simulink model "drm_simu"  (Simulink 8.6)
settings: Solver=VariableStepDiscrete  SolverMode=MultiTasking  StartTime=0.0  StopTime=12  RelTol=1e-3
PostLoadFcn:
  | init_drm
values from neighbouring files (symbols this model uses):
  sCRC_poly = struct(     'G16' ,{[1 0 0 0 1 0 0 0 0 0 0 1 0 0 0 0 1] ones(1,16)},     'G8'  ,{[1 0 0 0 1 1 1 0 1] ones(1,8)},     'G6'  ,{[1 1 0 1 1 1 1] ones(1,6)},     'G5'  ,{[1 1 0 1 1 1] ones(1,5)},     'G3'  ,{[1 0 1 0] ones(1,3)},     'G2'  ,{[1 1 1] ones(1,2)},     'G1'  ,{[1 1] 1} )    [crc_poly.m]
undefined symbols (not defined in the file or in its folder): channel, dfilt, fac, get, hot, if_mod, jet, magnitude, msc, ofdm, scrambler, sdc, sFFT, sync
libraries: dspmtrx3 x11, dspstat3 x7, commseqgen2 x6, dspobslib x6, dspsigops x5, commblkintrlv2 x4, dspsrcs4 x4, commsink2 x3, commrandsrc2 x3, commcrc2 x2, commcnvcod2 x2, commsequence2 x2
(part 1 of 2)
settings Model: Creator=Kevin Döring  LastModifiedBy=dtdsv
settings DataIOCC: LimitDataPoints=off  SaveOutput=off  SignalLogging=off  SaveTime=off
settings OptimizationCC: SimCompilerOptimization=on
settings DebuggingCC: InheritedTsInSrcMsg=none  MultiTaskCondExecSysMsg=none  MultiTaskRateTransMsg=warning  FcnCallInpInsideContextMsg=UseLocalSettings  FrameProcessingCompatibilityMsg=none
settings GRTTargetCC: GeneratePreprocessorConditionals=Use local settings

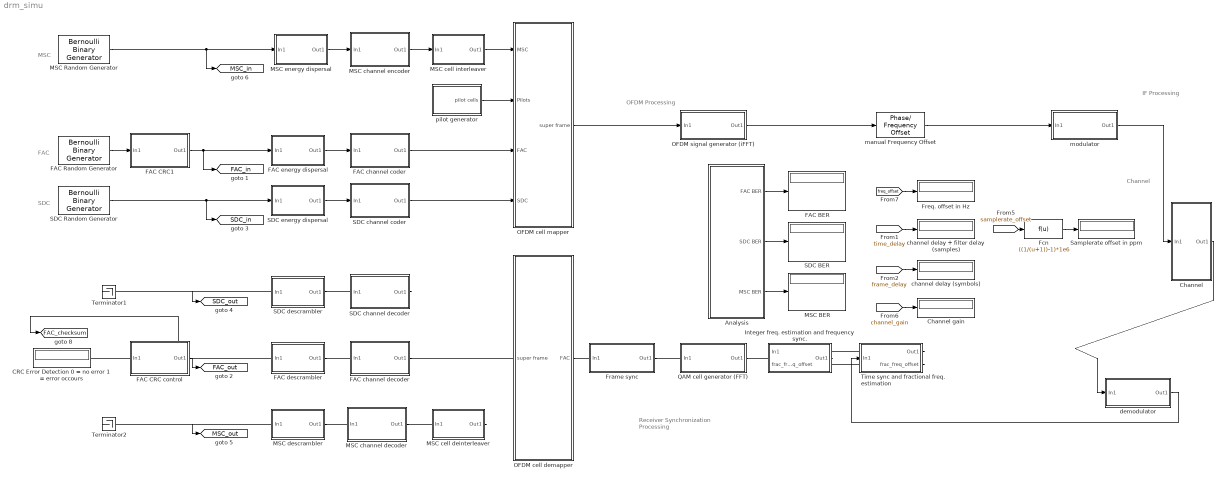
== system drm_simu ==
  note: FAC
  note: SDC
  note: MSC
  note: Receiver
      | Synchronization
      | Processing
  note: IF
      | Processing
  note: OFDM
      | Processing
  note: Channel
  Analysis : Subsystem
  CRC Error Detection 0 = no error 1 = error occours : Display
  Channel : Subsystem
  Channel gain : Display
  FAC BER : Display
  FAC CRC control : Subsystem
  FAC CRC1 : Subsystem
  FAC Random Generator : commrandsrc2/Bernoulli Binary Generator  P=0.5  seed=61  Ts=-1  frameBased=on  sampPerFrame=fac.Nmb_input_bits-8  orient=off  outDataType=double
  FAC channel coder : Subsystem
  FAC channel decoder : Subsystem
  FAC descrambler : Subsystem
  FAC energy dispersal : Subsystem
  Fcn : Fcn  Expr=((1/(u+1))-1)*1e6
  Frame sync : Subsystem
  Freq. offset in Hz : Display
  Integer freq. estimation and frequency sync. : Subsystem
  MSC BER : Display
  MSC Random Generator : commrandsrc2/Bernoulli Binary Generator  P=0.5  seed=61  Ts=sFFT.input_samplerate  frameBased=on  sampPerFrame=msc.Nmb_input_bits  orient=off  outDataType=double
  MSC cell deinterleaver : Subsystem
  MSC cell interleaver : Subsystem
  MSC channel decoder : Subsystem  BlockChoice=4QAM
      settings: AttributesFormatString=%<BlockChoice>  TemplateBlock=MSC_decoder_lib/MSC channel decoder  MemberBlocks=16QAM,4QAM,64QAM
  MSC channel encoder : Subsystem  BlockChoice=4QAM
      settings: AttributesFormatString=%<BlockChoice>  TemplateBlock=MSC_coder_lib/MSC channel encoder  MemberBlocks=16QAM,4QAM,64QAM
  MSC descrambler : Subsystem
  MSC energy dispersal : Subsystem
  OFDM cell demapper : Subsystem
  OFDM cell mapper : Subsystem
  OFDM signal generator (iFFT) : Subsystem
  QAM cell generator (FFT) : Subsystem
  SDC BER : Display
  SDC Random Generator : commrandsrc2/Bernoulli Binary Generator  P=0.5  seed=61  Ts=-1  frameBased=on  sampPerFrame=sdc.Nmb_input_bits  orient=off  outDataType=double
  SDC channel coder : Subsystem  BlockChoice=4QAM
      settings: AttributesFormatString=%<BlockChoice>  TemplateBlock=SDC_coder_lib/SDC channel coder  MemberBlocks=16QAM,4QAM
  SDC channel decoder : Subsystem  BlockChoice=4QAM
      settings: AttributesFormatString=%<BlockChoice>  TemplateBlock=SDC_decoder_lib/SDC channel decoder  MemberBlocks=16QAM,4QAM
  SDC descrambler : Subsystem
  SDC energy dispersal : Subsystem
  Samplerate offset in ppm : Display
  Terminator1 : Terminator
  Terminator2 : Terminator
  Time sync and fractional freq. estimation : Subsystem
  channel delay (symbols) : Display
  channel delay + filter delay (samples) : Display
  demodulator : Subsystem
  manual Frequency Offset : commrflib2/Phase// Frequency Offset  phaseOffset=0  freqPort=off  freqOffset=0
  modulator : Subsystem
  pilot generator : Subsystem
  tag scope: FAC_checksum=global, FAC_in=global, FAC_out=global, MSC_in=global, MSC_out=global, SDC_in=global, SDC_out=global
  wires:
  FAC Random Generator/1 -> FAC CRC1/1(In1)
  FAC energy dispersal/1(Out1) -> FAC channel coder/1(In1)
  FAC descrambler/1(Out1) -> [FAC_out], FAC CRC control/1(In1)
  FAC CRC1/1(Out1) -> FAC energy dispersal/1(In1), [FAC_in]
  FAC channel decoder/1(Out1) -> FAC descrambler/1(In1)
  FAC CRC control/1(Out1) -> CRC Error Detection 0 = no error 1 = error occours/1, [FAC_checksum]
  pilot generator/1(pilot cells) -> OFDM cell mapper/2(Pilots)
  SDC Random Generator/1 -> SDC energy dispersal/1(In1), [SDC_in]
  SDC energy dispersal/1(Out1) -> SDC channel coder/1(In1)
  SDC channel decoder/1(Out1) -> SDC descrambler/1(In1)
  SDC channel coder/1(Out1) -> OFDM cell mapper/4(SDC)
  SDC descrambler/1(Out1) -> [SDC_out], Terminator1/1
  FAC channel coder/1(Out1) -> OFDM cell mapper/3(FAC)
  ? -> SDC channel decoder/1(In1)
  MSC Random Generator/1 -> MSC energy dispersal/1(In1), [MSC_in]
  MSC channel encoder/1(Out1) -> MSC cell interleaver/1(In1)
  MSC energy dispersal/1(Out1) -> MSC channel encoder/1(In1)
  MSC cell interleaver/1(Out1) -> OFDM cell mapper/1(MSC)
  MSC channel decoder/1(Out1) -> MSC descrambler/1(In1)
  MSC cell deinterleaver/1(Out1) -> MSC channel decoder/1(In1)
  MSC descrambler/1(Out1) -> Terminator2/1, [MSC_out]
  ? -> MSC cell deinterleaver/1(In1)
  OFDM cell mapper/1(super frame) -> OFDM signal generator (iFFT)/1(In1)
  Analysis/2(SDC BER) -> SDC BER/1
  Analysis/3(MSC BER) -> MSC BER/1
  Analysis/1(FAC BER) -> FAC BER/1
  Frame sync/1(Out1) -> OFDM cell demapper/1(super frame)
  OFDM signal generator (iFFT)/1(Out1) -> manual Frequency Offset/1
  OFDM cell demapper/1(FAC) -> FAC channel decoder/1(In1)
  [freq_offset] -> Freq. offset in Hz/1
  [channel_gain] -> Channel gain/1
  [time_delay] -> channel delay + filter delay (samples)/1
  [frame_delay] -> channel delay (symbols)/1
  modulator/1(Out1) -> Channel/1(In1)
  [samplerate_offset] -> Fcn/1
  Fcn/1 -> Samplerate offset in ppm/1
  Time sync and fractional freq. estimation/1(Out1) -> Integer freq. estimation and frequency sync./1(In1)
  Integer freq. estimation and frequency sync./1(Out1) -> QAM cell generator (FFT)/1(In1)
  QAM cell generator (FFT)/1(Out1) -> Frame sync/1(In1)
  Time sync and fractional freq. estimation/2(frac_freq_offset) -> Integer freq. estimation and frequency sync./2(frac_freq_offset)
  demodulator/1(Out1) -> Time sync and fractional freq. estimation/1(In1)
  Channel/1(Out1) -> demodulator/1(In1)
  manual Frequency Offset/1 -> modulator/1(In1)

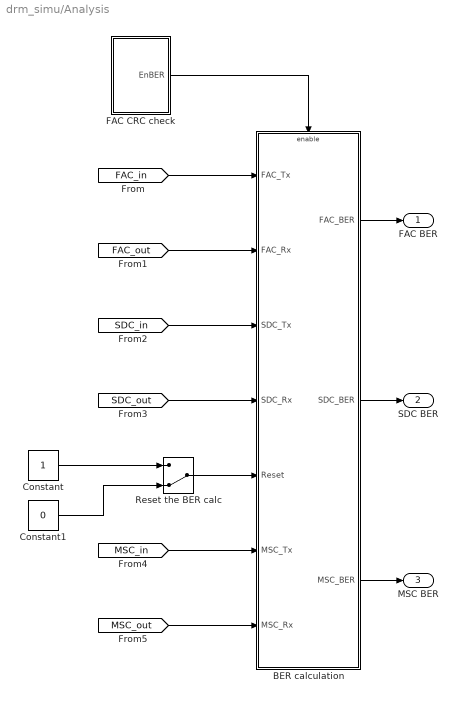
== system drm_simu/Analysis ==
  BER calculation : Subsystem
  Constant : Constant
  Constant1 : Constant  Value=0
  FAC CRC check : Subsystem
  Reset the BER calc : ManualSwitch  CurrentSetting=0
  FAC BER : Outport
  SDC BER : Outport  Port=2
  MSC BER : Outport  Port=3
  wires:
  [SDC_in] -> BER calculation/3(SDC_Tx)
  [SDC_out] -> BER calculation/4(SDC_Rx)
  [FAC_out] -> BER calculation/2(FAC_Rx)
  [FAC_in] -> BER calculation/1(FAC_Tx)
  [MSC_out] -> BER calculation/7(MSC_Rx)
  BER calculation/1(FAC_BER) -> FAC BER/1
  BER calculation/2(SDC_BER) -> SDC BER/1
  BER calculation/3(MSC_BER) -> MSC BER/1
  [MSC_in] -> BER calculation/6(MSC_Tx)
  Constant/1 -> Reset the BER calc/1
  Reset the BER calc/1 -> BER calculation/5(Reset)
  FAC CRC check/1(EnBER) -> BER calculation/Enable
  Constant1/1 -> Reset the BER calc/2

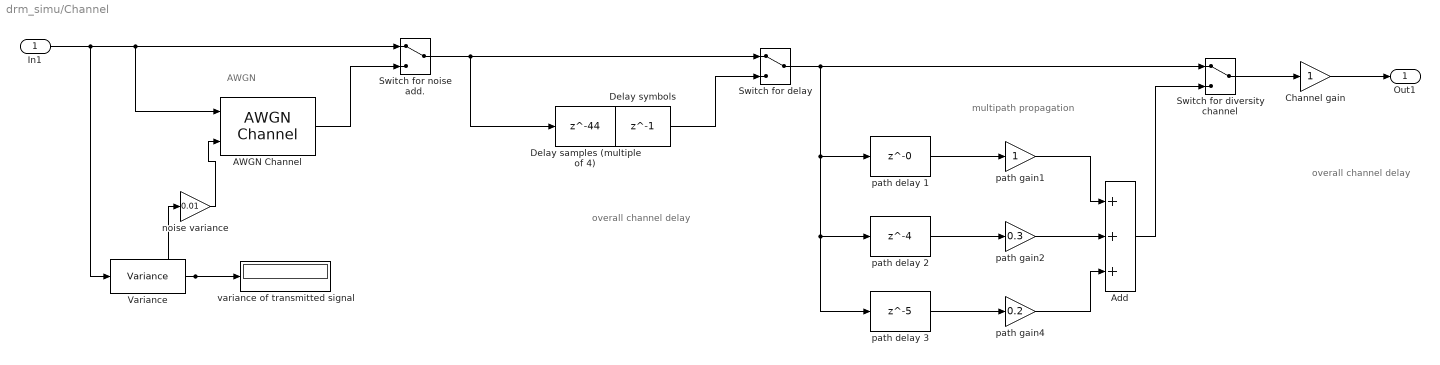
== system drm_simu/Channel ==
  note: AWGN
  note: overall channel
      | delay
  note: multipath
      | propagation
  note: overall channel
      | delay
  In1 : Inport
  AWGN Channel : commchan3/AWGN Channel  InputProcessing=Inherited (this choice will be removed - see release notes)  seed=67  noiseMode=Variance from port  EbNodB=10  EsNodB=10  SNRdB=10  bitsPerSym=1  Ps=1  Tsym=1  variance=1
  Add : Sum  Inputs=+++
  Channel gain : Gain
  Delay samples (multiple of 4) : Delay  DelayLength=44  InitialCondition=0  InputProcessing=Inherited
  Delay symbols : Delay  DelayLength=1  InitialCondition=0  InputProcessing=Inherited
  Switch for delay : ManualSwitch
  Switch for diversity channel : ManualSwitch
  Switch for noise add. : ManualSwitch
  Variance : dspstat3/Variance  run=off  reset_popup=None  InputProcessing=Columns as channels (frame based)  directionMode=Each column  dimension=1  roiEnable=off  roiType=Rectangles  roiPortion=Entire ROI  roiOutput=Individual statistics for each ROI  roiFlag=off  roundingMode=Floor  overflowMode=off
  noise variance : Gain  Gain=0.01
  path delay 1 : Delay  DelayLength=0  InitialCondition=0  InputProcessing=Inherited
  path delay 2 : Delay  DelayLength=4  InitialCondition=0  InputProcessing=Inherited
  path delay 3 : Delay  DelayLength=5  InitialCondition=0  InputProcessing=Inherited
  path gain1 : Gain
  path gain2 : Gain  Gain=0.3
  path gain4 : Gain  Gain=0.2
  variance of transmitted signal : Display
      settings: SampleTime=2^14
  Out1 : Outport
  wires:
  Variance/1 -> variance of transmitted signal/1, noise variance/1
  In1/1 -> Variance/1, Switch for noise add./1, AWGN Channel/1
  AWGN Channel/1 -> Switch for noise add./2
  Delay samples (multiple of 4)/1 -> Delay symbols/1
  Switch for noise add./1 -> Delay samples (multiple of 4)/1, Switch for delay/1
  Delay symbols/1 -> Switch for delay/2
  Channel gain/1 -> Out1/1
  noise variance/1 -> AWGN Channel/2
  Switch for diversity channel/1 -> Channel gain/1
  Switch for delay/1 -> path delay 1/1, path delay 2/1, path delay 3/1, Switch for diversity channel/1
  Add/1 -> Switch for diversity channel/2
  path delay 1/1 -> path gain1/1
  path delay 2/1 -> path gain2/1
  path gain2/1 -> Add/2
  path gain1/1 -> Add/1
  path delay 3/1 -> path gain4/1
  path gain4/1 -> Add/3

== system drm_simu/FAC CRC control ==
  In1 : Inport
  Data Type Conversion1 : DataTypeConversion  OutDataTypeStr=double
  General CRC Syndrome Detector : commcrc2/General CRC Syndrome Detector  genPoly=sCRC_poly(1).G8  iniStates=sCRC_poly(2).G8  directMethod=off  reflectInputBytes=off  reflectChecksums=off  finalXOR=0  numChecksums=1
  Logical Operator : Logic  Operator=NOT  AllPortsSameDT=off  OutDataTypeStr=boolean
  Submatrix : dspmtrx3/Submatrix  RowSpan=Range of rows  RowStartMode=First  RowStartIndex=1  RowEndMode=Index  RowEndIndex=fac.Nmb_input_bits-8  ColSpan=All columns  ColStartMode=First  ColStartIndex=1  ColEndMode=Index  ColEndIndex=64
  Submatrix1 : dspmtrx3/Submatrix  RowSpan=Range of rows  RowStartMode=Offset from last  RowStartIndex=length(sCRC_poly(2).G8)-1  RowEndMode=Last  RowEndIndex=64  ColSpan=All columns  ColStartMode=First  ColStartIndex=1  ColEndMode=Index  ColEndIndex=64
  Terminator : Terminator
  Vector Concatenate : Concatenate  Mode=Multidimensional array
  Out1 : Outport
  wires:
  Submatrix/1 -> Vector Concatenate/1
  Submatrix1/1 -> Logical Operator/1
  Data Type Conversion1/1 -> Vector Concatenate/2
  Logical Operator/1 -> Data Type Conversion1/1
  Vector Concatenate/1 -> General CRC Syndrome Detector/1
  General CRC Syndrome Detector/2 -> Out1/1
  General CRC Syndrome Detector/1 -> Terminator/1
  In1/1 -> Submatrix/1, Submatrix1/1

== system drm_simu/FAC CRC1 ==
  In1 : Inport
  Data Type Conversion1 : DataTypeConversion  OutDataTypeStr=double
  FAC CRC : commcrc2/General CRC Generator  genPoly=sCRC_poly(1).G8  iniStates=sCRC_poly(2).G8  directMethod=off  reflectInputBytes=off  reflectChecksums=off  finalXOR=0  numChecksums=1
  Logical Operator : Logic  Operator=NOT  AllPortsSameDT=off  OutDataTypeStr=boolean
  Submatrix : dspmtrx3/Submatrix  RowSpan=Range of rows  RowStartMode=First  RowStartIndex=1  RowEndMode=Index  RowEndIndex=fac.Nmb_input_bits-8  ColSpan=All columns  ColStartMode=First  ColStartIndex=1  ColEndMode=Index  ColEndIndex=64
  Submatrix1 : dspmtrx3/Submatrix  RowSpan=Range of rows  RowStartMode=Offset from last  RowStartIndex=length(sCRC_poly(2).G8)-1  RowEndMode=Last  RowEndIndex=64  ColSpan=All columns  ColStartMode=First  ColStartIndex=1  ColEndMode=Index  ColEndIndex=64
  Vector Concatenate : Concatenate  Mode=Multidimensional array
  Out1 : Outport
  wires:
  FAC CRC/1 -> Submatrix/1, Submatrix1/1
  Submatrix/1 -> Vector Concatenate/1
  Submatrix1/1 -> Logical Operator/1
  Data Type Conversion1/1 -> Vector Concatenate/2
  Logical Operator/1 -> Data Type Conversion1/1
  In1/1 -> FAC CRC/1
  Vector Concatenate/1 -> Out1/1

== system drm_simu/FAC channel coder ==
  In1 : Inport
  Bit interleaver : commblkintrlv2/General Block Interleaver  permutationVectorSource=Dialog  elements=fac.interleave_P0
  Encoder : Subsystem
  Rectangular QAM Modulator Baseband : commdigbbndam3/Rectangular QAM Modulator Baseband  M=FAC_QAM  InType=Bit  Enc=User-defined  Mapping=fac.qam_map  PowType=Min. distance between symbols  MinDist=fac.qam_norm  AvgPow=2  PeakPow=1  Ph=0  outDtype=double  outWordLen=16  outUDDataType=sfix(16)  outFracLenMode=Best precision  outFracLen=15
  Out1 : Outport
  wires:
  Encoder/1(Out1) -> Bit interleaver/1
  Bit interleaver/1 -> Rectangular QAM Modulator Baseband/1
  In1/1 -> Encoder/1(In1)
  Rectangular QAM Modulator Baseband/1 -> Out1/1

== system drm_simu/FAC channel decoder ==
  In1 : Inport
  Decoder : Subsystem
  General Block Deinterleaver : commblkintrlv2/General Block Deinterleaver  permutationVectorSource=Dialog  elements=fac.interleave_P0
  Rectangular QAM Demodulator Baseband : commdigbbndam3/Rectangular QAM Demodulator Baseband  M=FAC_QAM  PowType=Min. distance between symbols  MinDist=fac.qam_norm  AvgPow=1  PeakPow=1  Ph=0  Dec=User-defined  Mapping=fac.qam_map  OutType=Bit  DecType=Hard decision  VarSource=Dialog  Variance=1  outDtype1=Inherit via internal rule  outDtype2=Inherit via internal rule  derotateFactorWordLen=16  denormFactorWordLen=16  prodOutWordLen=32  prodOutRoundingMode=Floor  prodOutOverflowMode=Wrap  sumWordLen=32
  Out1 : Outport
  wires:
  Rectangular QAM Demodulator Baseband/1 -> General Block Deinterleaver/1
  General Block Deinterleaver/1 -> Decoder/1(In1)
  Decoder/1(Out1) -> Out1/1
  In1/1 -> Rectangular QAM Demodulator Baseband/1

== system drm_simu/FAC descrambler ==
  In1 : Inport
  Constant : Constant  Value=scrambler.fac.reset_vec  VectorParams1D=off  SampleTime=2505/72  FramePeriod=scrambler.fac.res_samplerate
      settings: SamplingMode=Frame based
  Data Type Conversion : DataTypeConversion  OutDataTypeStr=double
  Data Type Conversion1 : DataTypeConversion  OutDataTypeStr=boolean
  Frame Conversion : FrameConversion  InheritSamplingMode=off
  Logical Operator : Logic  Operator=XOR  AllPortsSameDT=off  OutDataTypeStr=boolean
  PN Sequence Generator : commseqgen2/PN Sequence Generator  poly=scrambler.poly  ini_sta=scrambler.init  outBitMaskSource=Dialog parameter  shift=9  outVarSiz=off  maxOutSizeMode=Dialog parameter  maxOutSize=[10 1]  Ts=scrambler.fac.pn_samplerate  frameBased=on  sampPerFrame=fac.Nmb_input_bits  reset=on  bitPackedOutputs=off  outDataType=boolean  numPackedBits=8  bitPackDataSigned=off  bitPackedOutDType=double
  Out1 : Outport
  wires:
  Logical Operator/1 -> Data Type Conversion/1
  PN Sequence Generator/1 -> Logical Operator/1
  Constant/1 -> PN Sequence Generator/1
  Frame Conversion/1 -> Out1/1
  Data Type Conversion/1 -> Frame Conversion/1
  Data Type Conversion1/1 -> Logical Operator/2
  In1/1 -> Data Type Conversion1/1

== system drm_simu/FAC energy dispersal ==
  In1 : Inport
  Constant : Constant  Value=scrambler.fac.reset_vec  VectorParams1D=off  SampleTime=2505/72  FramePeriod=scrambler.fac.res_samplerate
      settings: SamplingMode=Frame based
  Data Type Conversion : DataTypeConversion  OutDataTypeStr=double
  Data Type Conversion1 : DataTypeConversion  OutDataTypeStr=boolean
  Frame Conversion : FrameConversion  InheritSamplingMode=off
  Logical Operator : Logic  Operator=XOR  AllPortsSameDT=off  OutDataTypeStr=boolean
  PN Sequence Generator : commseqgen2/PN Sequence Generator  poly=scrambler.poly  ini_sta=scrambler.init  outBitMaskSource=Dialog parameter  shift=9  outVarSiz=off  maxOutSizeMode=Dialog parameter  maxOutSize=[10 1]  Ts=scrambler.fac.pn_samplerate  frameBased=on  sampPerFrame=fac.Nmb_input_bits  reset=on  bitPackedOutputs=off  outDataType=boolean  numPackedBits=8  bitPackDataSigned=off  bitPackedOutDType=double
  Out1 : Outport
  wires:
  Logical Operator/1 -> Data Type Conversion/1
  PN Sequence Generator/1 -> Logical Operator/1
  Constant/1 -> PN Sequence Generator/1
  Frame Conversion/1 -> Out1/1
  Data Type Conversion/1 -> Frame Conversion/1
  Data Type Conversion1/1 -> Logical Operator/2
  In1/1 -> Data Type Conversion1/1

== system drm_simu/Frame sync ==
  In1 : Inport
  Add : Sum  Inputs=+-
  Frame Sync : Subsystem
  Frame timing : Scope
  Variable Integer Delay : dspobslib/Variable Integer Delay  dmax=ofdm.nmb_carriers*ofdm.nmb_symbols*ofdm.superframe_size  InputProcessing=Inherited (this choice will be removed - see release notes)  ic=0  noDFT=off
  nmb_carriers : Gain  Gain=ofdm.nmb_carriers
  ofdm superframe : Constant  Value=ofdm.nmb_carriers*ofdm.nmb_symbols*ofdm.superframe_size
  sub. 1 because one symbol delay is for time sync. : Fcn  Expr=u-1
  Out1 : Outport
  tag scope: frame_delay=global
  wires:
  In1/1 -> Variable Integer Delay/1, Frame Sync/1(In1)
  Variable Integer Delay/1 -> Out1/1
  Frame Sync/1(Frame timing) -> nmb_carriers/1, sub. 1 because one symbol delay is for time sync./1
  Add/1 -> Variable Integer Delay/2
  nmb_carriers/1 -> Add/2
  ofdm superframe/1 -> Add/1
  sub. 1 because one symbol delay is for time sync./1 -> [frame_delay]
  Frame Sync/2(Frame timing signal) -> Frame timing/1

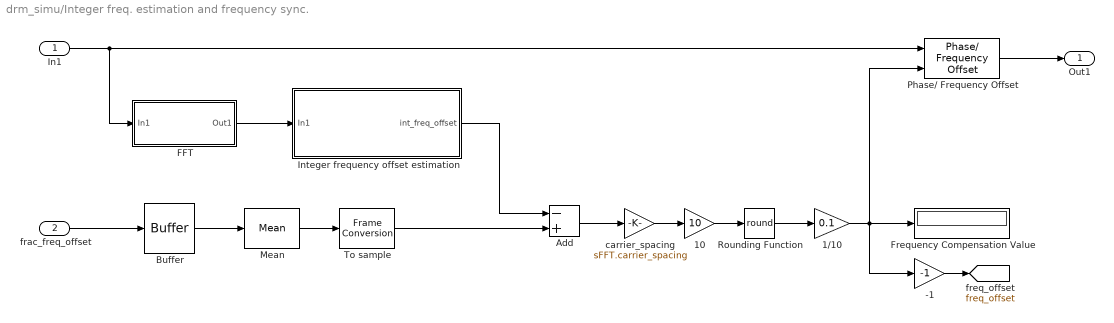
== system drm_simu/Integer freq. estimation and frequency sync. ==
  In1 : Inport
  frac_freq_offset : Inport  Port=2
  -1 : Gain  Gain=-1
  1/10 : Gain  Gain=0.1
  10 : Gain  Gain=10
  Add : Sum  Inputs=-+
  Buffer : Buffer  N=ofdm.nmb_symbols
  FFT : Subsystem
  Frequency Compensation Value : Display
  Integer frequency offset estimation : Subsystem
  Mean : dspstat3/Mean  run=off  reset_popup=None  InputProcessing=Columns as channels (frame based)  directionMode=Each column  dimension=1  roiEnable=off  roiType=Rectangles  roiPortion=Entire ROI  roiOutput=Individual statistics for each ROI  roiFlag=off  outputDataTypeStr=Inherit: Same as accumulator  outputLastDataTypeStr=Inherit: Same as accumulator  outputMin=[]  outputMax=[]  roundingMode=Floor  overflowMode=off
  Phase/ Frequency Offset : commrflib2/Phase// Frequency Offset  phaseOffset=0  freqPort=on  freqOffset=0
  Rounding Function : Rounding  Operator=round
  To sample : FrameConversion  InheritSamplingMode=off  OutFrame=Sample-based
  carrier_spacing : Gain  Gain=sFFT.carrier_spacing
  Out1 : Outport
  tag scope: freq_offset=global
  wires:
  In1/1 -> Phase/ Frequency Offset/1, FFT/1(In1)
  Phase/ Frequency Offset/1 -> Out1/1
  -1/1 -> [freq_offset]
  FFT/1(Out1) -> Integer frequency offset estimation/1(In1)
  frac_freq_offset/1 -> Buffer/1
  Buffer/1 -> Mean/1
  Mean/1 -> To sample/1
  10/1 -> Rounding Function/1
  Rounding Function/1 -> 1/10/1
  carrier_spacing/1 -> 10/1
  1/10/1 -> Frequency Compensation Value/1, -1/1, Phase/ Frequency Offset/2
  Add/1 -> carrier_spacing/1
  Integer frequency offset estimation/1(int_freq_offset) -> Add/1
  To sample/1 -> Add/2

== system drm_simu/MSC cell deinterleaver ==
  In1 : Inport
  General Multiplexed Deinterleaver : commcnvintrlv2/General Multiplexed Deinterleaver  delay=msc.long_interleave_vec  ic=0
  short deinterleaving : commblkintrlv2/General Block Deinterleaver  permutationVectorSource=Dialog  elements=msc.cell_interleave_P
  Out1 : Outport
  wires:
  In1/1 -> General Multiplexed Deinterleaver/1
  short deinterleaving/1 -> Out1/1
  General Multiplexed Deinterleaver/1 -> short deinterleaving/1

== system drm_simu/MSC cell interleaver ==
  In1 : Inport
  General Multiplexed Interleaver : commcnvintrlv2/General Multiplexed Interleaver  delay=msc.long_interleave_vec  ic=0
  short interleaving : commblkintrlv2/General Block Interleaver  permutationVectorSource=Dialog  elements=msc.cell_interleave_P
  Out1 : Outport
  wires:
  short interleaving/1 -> General Multiplexed Interleaver/1
  General Multiplexed Interleaver/1 -> Out1/1
  In1/1 -> short interleaving/1

== system drm_simu/MSC channel decoder ==
  In1 : Inport
  4QAM : MSC_decoder_lib/4QAM
  Out1 : Outport
  wires:
  In1/1 -> 4QAM/1
  4QAM/1 -> Out1/1

== system drm_simu/MSC channel encoder ==
  In1 : Inport
  4QAM : MSC_coder_lib/4QAM
  Out1 : Outport
  wires:
  In1/1 -> 4QAM/1
  4QAM/1 -> Out1/1

== system drm_simu/MSC descrambler ==
  In1 : Inport
  Constant : Constant  Value=scrambler.msc.reset_vec  VectorParams1D=off  SampleTime=2505/72  FramePeriod=scrambler.msc.res_samplerate
      settings: SamplingMode=Frame based
  Data Type Conversion : DataTypeConversion  OutDataTypeStr=double
  Data Type Conversion1 : DataTypeConversion  OutDataTypeStr=boolean
  Frame Conversion : FrameConversion  InheritSamplingMode=off
  Logical Operator : Logic  Operator=XOR  AllPortsSameDT=off  OutDataTypeStr=boolean
  PN Sequence Generator : commseqgen2/PN Sequence Generator  poly=scrambler.poly  ini_sta=scrambler.init  outBitMaskSource=Dialog parameter  shift=9  outVarSiz=off  maxOutSizeMode=Dialog parameter  maxOutSize=[10 1]  Ts=scrambler.msc.pn_samplerate  frameBased=on  sampPerFrame=msc.Nmb_input_bits  reset=on  bitPackedOutputs=off  outDataType=boolean  numPackedBits=8  bitPackDataSigned=off  bitPackedOutDType=double
  Out1 : Outport
  wires:
  In1/1 -> Data Type Conversion1/1
  Data Type Conversion1/1 -> Logical Operator/2
  Data Type Conversion/1 -> Frame Conversion/1
  Frame Conversion/1 -> Out1/1
  Constant/1 -> PN Sequence Generator/1
  PN Sequence Generator/1 -> Logical Operator/1
  Logical Operator/1 -> Data Type Conversion/1

== system drm_simu/MSC energy dispersal ==
  In1 : Inport
  Constant : Constant  Value=scrambler.msc.reset_vec  VectorParams1D=off  SampleTime=2505/72  FramePeriod=scrambler.msc.res_samplerate
      settings: SamplingMode=Frame based
  Data Type Conversion : DataTypeConversion  OutDataTypeStr=double
  Data Type Conversion1 : DataTypeConversion  OutDataTypeStr=boolean
  Frame Conversion : FrameConversion  InheritSamplingMode=off
  Logical Operator : Logic  Operator=XOR  AllPortsSameDT=off  OutDataTypeStr=boolean
  PN Sequence Generator : commseqgen2/PN Sequence Generator  poly=scrambler.poly  ini_sta=scrambler.init  outBitMaskSource=Dialog parameter  shift=9  outVarSiz=off  maxOutSizeMode=Dialog parameter  maxOutSize=[10 1]  Ts=scrambler.msc.pn_samplerate  frameBased=on  sampPerFrame=msc.Nmb_input_bits  reset=on  bitPackedOutputs=off  outDataType=boolean  numPackedBits=8  bitPackDataSigned=off  bitPackedOutDType=double
  Out1 : Outport
  wires:
  In1/1 -> Data Type Conversion1/1
  Data Type Conversion1/1 -> Logical Operator/2
  Data Type Conversion/1 -> Frame Conversion/1
  Frame Conversion/1 -> Out1/1
  Constant/1 -> PN Sequence Generator/1
  PN Sequence Generator/1 -> Logical Operator/1
  Logical Operator/1 -> Data Type Conversion/1

== system drm_simu/OFDM cell demapper ==
  super frame : Inport
  Channel estimation and compensation : Subsystem
  Discrete-Time Scatter Plot Scope : ConstellationDiagram  Tag=ScatterPlot
  FAC cell selector : Selector  InputPortWidth=ofdm.nmb_carriers*ofdm.nmb_symbols  IndexOptions=Index vector (dialog)  Indices=ofdm.FAC_cell_index  OutputSizes=1
  MER measurment : Subsystem
  MER/dB : Display
  Rebuffer superframe to frames : Buffer  N=ofdm.nmb_carriers*ofdm.nmb_symbols
  collect one superframe : Buffer  N=ofdm.nmb_carriers*ofdm.superframe_size*ofdm.nmb_symbols
  FAC : Outport
  wires:
  super frame/1 -> collect one superframe/1
  Rebuffer superframe to frames/1 -> FAC cell selector/1
  collect one superframe/1 -> Channel estimation and compensation/1(In1)
  Channel estimation and compensation/1(Out1) -> Rebuffer superframe to frames/1
  FAC cell selector/1 -> FAC/1, MER measurment/1(In1), Discrete-Time Scatter Plot Scope/1
  MER measurment/1(MER) -> MER/dB/1

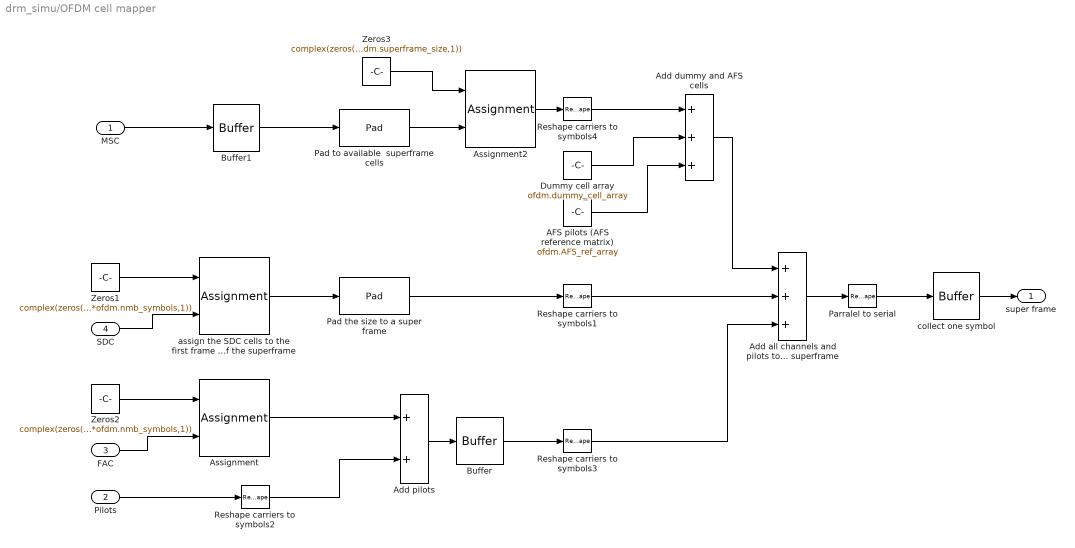
== system drm_simu/OFDM cell mapper ==
  MSC : Inport
  Pilots : Inport  Port=2
  FAC : Inport  Port=3
  SDC : Inport  Port=4
  AFS pilots (AFS reference matrix) : Constant  Value=ofdm.AFS_ref_array  VectorParams1D=off
      settings: SamplingMode=Frame based
  Add all channels and pilots to OFDM superframe : Sum  Inputs=+++
  "Add dummy and AFS cells " : Sum  Inputs=+++
  Add pilots : Sum
  Assignment : Assignment  OutputInitialize=Specify size for each dimension in table  IndexOptions=Index vector (dialog)  Indices=ofdm.FAC_cell_index  OutputSizes=102
  Assignment2 : Assignment  OutputInitialize=Specify size for each dimension in table  IndexOptions=Index vector (dialog)  Indices=ofdm.MSC_cell_index  OutputSizes=102
  Buffer : Buffer  N=ofdm.nmb_carriers*ofdm.nmb_symbols*ofdm.superframe_size
  Buffer1 : Buffer  N=ofdm.superframe_size*msc.NmbQAMcells
  Dummy cell array : Constant  Value=ofdm.dummy_cell_array  VectorParams1D=off
      settings: SamplingMode=Frame based
  Pad the size to a super frame : dspsigops/Pad  padAlong=Columns  dimsToPad=1  valSrc=Specify via dialog  padVal=0  spec=Output size  padNumOutRowsSpecMethod=User-specified  numOutRows=ofdm.nmb_carriers*ofdm.nmb_symbols*ofdm.superframe_size  padNumOutColsSpecMethod=User-specified  numOutCols=3*ofdm.nmb_carriers*ofdm.nmb_symbols  isVarDimsMode=off  padBeginning=0  padEnd=0  outSizeMode=User-specified  outSize=1  padSigAt=End  trunc_flag=None  roundingMode=Floor  overflowMode=off  truncOrWrapMode=Truncate  wrap_flag=None
  Pad to available  superframe cells : dspsigops/Pad  padAlong=Columns  dimsToPad=1  valSrc=Specify via dialog  padVal=0  spec=Output size  padNumOutRowsSpecMethod=User-specified  numOutRows=ofdm.Nmb_MSC_cells  padNumOutColsSpecMethod=User-specified  numOutCols=3*ofdm.nmb_carriers*ofdm.nmb_symbols  isVarDimsMode=off  padBeginning=0  padEnd=0  outSizeMode=User-specified  outSize=1  padSigAt=End  trunc_flag=None  roundingMode=Floor  overflowMode=off  truncOrWrapMode=Truncate  wrap_flag=None
  Parralel to serial : Reshape  OutputDimensionality=Column vector (2-D)
  Reshape carriers to symbols1 : Reshape  OutputDimensionality=Customize  OutputDimensions=[ofdm.nmb_carriers,ofdm.superframe_size*ofdm.nmb_symbols]
  Reshape carriers to symbols2 : Reshape  OutputDimensionality=Column vector (2-D)  OutputDimensions=[ofdm.nmb_carriers,ofdm.superframe_size*ofdm.nmb_symbols]
  Reshape carriers to symbols3 : Reshape  OutputDimensionality=Customize  OutputDimensions=[ofdm.nmb_carriers,ofdm.superframe_size*ofdm.nmb_symbols]
  Reshape carriers to symbols4 : Reshape  OutputDimensionality=Customize  OutputDimensions=[ofdm.nmb_carriers,ofdm.superframe_size*ofdm.nmb_symbols]
  Zeros1 : Constant  Value=complex(zeros(ofdm.nmb_carriers*ofdm.nmb_symbols,1))  VectorParams1D=off
      settings: SamplingMode=Frame based
  Zeros2 : Constant  Value=complex(zeros(ofdm.nmb_carriers*ofdm.nmb_symbols,1))  VectorParams1D=off
      settings: SamplingMode=Frame based
  Zeros3 : Constant  Value=complex(zeros(ofdm.nmb_carriers*ofdm.nmb_symbols*ofdm.superframe_size,1))  VectorParams1D=off
      settings: SamplingMode=Frame based
  assign the SDC cells to the first frame of the superframe : Assignment  OutputInitialize=Specify size for each dimension in table  IndexOptions=Index vector (dialog)  Indices=ofdm.SDC_cell_index  OutputSizes=102
  collect one symbol : Buffer  N=ofdm.nmb_carriers
  super frame : Outport
  wires:
  Zeros2/1 -> Assignment/1
  SDC/1 -> assign the SDC cells to the first frame of the superframe/2
  assign the SDC cells to the first frame of the superframe/1 -> Pad the size to a super frame/1
  Reshape carriers to symbols1/1 -> Add all channels and pilots to OFDM superframe/2
  Zeros1/1 -> assign the SDC cells to the first frame of the superframe/1
  Pad the size to a super frame/1 -> Reshape carriers to symbols1/1
  MSC/1 -> Buffer1/1
  Buffer1/1 -> Pad to available  superframe cells/1
  Assignment2/1 -> Reshape carriers to symbols4/1
  Pad to available  superframe cells/1 -> Assignment2/2
  Zeros3/1 -> Assignment2/1
  Reshape carriers to symbols4/1 -> "Add dummy and AFS cells "/1
  "Add dummy and AFS cells "/1 -> Add all channels and pilots to OFDM superframe/1
  Dummy cell array/1 -> "Add dummy and AFS cells "/2
  Reshape carriers to symbols3/1 -> Add all channels and pilots to OFDM superframe/3
  FAC/1 -> Assignment/2
  Buffer/1 -> Reshape carriers to symbols3/1
  Add all channels and pilots to OFDM superframe/1 -> Parralel to serial/1
  Assignment/1 -> Add pilots/1
  Pilots/1 -> Reshape carriers to symbols2/1
  Add pilots/1 -> Buffer/1
  Reshape carriers to symbols2/1 -> Add pilots/2
  AFS pilots (AFS reference matrix)/1 -> "Add dummy and AFS cells "/3
  collect one symbol/1 -> super frame/1
  Parralel to serial/1 -> collect one symbol/1

== system drm_simu/OFDM signal generator (iFFT) ==
  In1 : Inport
  Append guard interval : Selector  NumberOfDimensions=2  InputPortWidth=3  IndexOptions=Index vector (dialog),Select all  Indices=sFFT.guard_index,1  OutputSizes=1,1
  IFFT : MATLABFcn  MATLABFcn=ifft  Output1D=off
  Pad to FFT size : dspsigops/Pad  padAlong=Columns  dimsToPad=1  valSrc=Specify via dialog  padVal=0  spec=Output size  padNumOutRowsSpecMethod=User-specified  numOutRows=sFFT.size  padNumOutColsSpecMethod=User-specified  numOutCols=1  isVarDimsMode=off  padBeginning=0  padEnd=0  outSizeMode=User-specified  outSize=1  padSigAt=End  trunc_flag=None  roundingMode=Floor  overflowMode=off  truncOrWrapMode=Truncate  wrap_flag=None
  Pad to complete symbol size (useful part + guard) : dspsigops/Pad  padAlong=Columns  dimsToPad=1  valSrc=Specify via dialog  padVal=0  spec=Output size  padNumOutRowsSpecMethod=User-specified  numOutRows=sFFT.symbol_length  padNumOutColsSpecMethod=User-specified  numOutCols=1  isVarDimsMode=off  padBeginning=0  padEnd=0  outSizeMode=User-specified  outSize=1  padSigAt=End  trunc_flag=None  roundingMode=Floor  overflowMode=off  truncOrWrapMode=Truncate  wrap_flag=None
  Shift carriers for ifft : Selector  NumberOfDimensions=2  InputPortWidth=3  IndexOptions=Index vector (dialog),Select all  Indices=sFFT.shift_vec,1  OutputSizes=1,1
  Out1 : Outport
  wires:
  In1/1 -> Pad to FFT size/1
  IFFT/1 -> Pad to complete symbol size (useful part + guard)/1
  Pad to FFT size/1 -> Shift carriers for ifft/1
  Shift carriers for ifft/1 -> IFFT/1
  Append guard interval/1 -> Out1/1
  Pad to complete symbol size (useful part + guard)/1 -> Append guard interval/1

== system drm_simu/QAM cell generator (FFT) ==
  In1 : Inport
  FFT : MATLABFcn  MATLABFcn=fft  Output1D=off
  Rebuild number of carriers : dspmtrx3/Submatrix  RowSpan=Range of rows  RowStartMode=First  RowStartIndex=1  RowEndMode=Index  RowEndIndex=ofdm.nmb_carriers  ColSpan=All columns  ColStartMode=First  ColStartIndex=1  ColEndMode=Last  ColEndIndex=1
  Remove guard interval : dspmtrx3/Submatrix  RowSpan=Range of rows  RowStartMode=Index  RowStartIndex=sFFT.guard_size+1  RowEndMode=Last  RowEndIndex=sFFT.symbol_length  ColSpan=All columns  ColStartMode=First  ColStartIndex=1  ColEndMode=Last  ColEndIndex=1
  Shift back carriers : Selector  NumberOfDimensions=2  InputPortWidth=3  IndexOptions=Index vector (dialog),Select all  Indices=sFFT.backshift_vec,1  OutputSizes=1,1
  Out1 : Outport
  wires:
  FFT/1 -> Shift back carriers/1
  Shift back carriers/1 -> Rebuild number of carriers/1
  Remove guard interval/1 -> FFT/1
  Rebuild number of carriers/1 -> Out1/1
  In1/1 -> Remove guard interval/1

== system drm_simu/SDC channel coder ==
  In1 : Inport
  4QAM : SDC_coder_lib/4QAM
  Out1 : Outport
  wires:
  In1/1 -> 4QAM/1
  4QAM/1 -> Out1/1

== system drm_simu/SDC channel decoder ==
  In1 : Inport
  4QAM : SDC_decoder_lib/4QAM
  Out1 : Outport
  wires:
  In1/1 -> 4QAM/1
  4QAM/1 -> Out1/1

== system drm_simu/SDC descrambler ==
  In1 : Inport
  Constant : Constant  Value=scrambler.sdc.reset_vec  VectorParams1D=off  SampleTime=2505/72  FramePeriod=scrambler.sdc.res_samplerate
      settings: SamplingMode=Frame based
  Data Type Conversion : DataTypeConversion  OutDataTypeStr=double
  Data Type Conversion1 : DataTypeConversion  OutDataTypeStr=boolean
  Frame Conversion : FrameConversion  InheritSamplingMode=off
  Logical Operator : Logic  Operator=XOR  AllPortsSameDT=off  OutDataTypeStr=boolean
  PN Sequence Generator : commseqgen2/PN Sequence Generator  poly=scrambler.poly  ini_sta=scrambler.init  outBitMaskSource=Dialog parameter  shift=9  outVarSiz=off  maxOutSizeMode=Dialog parameter  maxOutSize=[10 1]  Ts=scrambler.sdc.pn_samplerate  frameBased=on  sampPerFrame=sdc.Nmb_input_bits  reset=on  bitPackedOutputs=off  outDataType=boolean  numPackedBits=8  bitPackDataSigned=off  bitPackedOutDType=double
  Out1 : Outport
  wires:
  In1/1 -> Data Type Conversion1/1
  Data Type Conversion1/1 -> Logical Operator/2
  Data Type Conversion/1 -> Frame Conversion/1
  Frame Conversion/1 -> Out1/1
  Constant/1 -> PN Sequence Generator/1
  PN Sequence Generator/1 -> Logical Operator/1
  Logical Operator/1 -> Data Type Conversion/1

== system drm_simu/SDC energy dispersal ==
  In1 : Inport
  Constant : Constant  Value=scrambler.sdc.reset_vec  VectorParams1D=off  SampleTime=2505/72  FramePeriod=scrambler.sdc.res_samplerate
      settings: SamplingMode=Frame based
  Data Type Conversion : DataTypeConversion  OutDataTypeStr=double
  Data Type Conversion1 : DataTypeConversion  OutDataTypeStr=boolean
  Frame Conversion : FrameConversion  InheritSamplingMode=off
  Logical Operator : Logic  Operator=XOR  AllPortsSameDT=off  OutDataTypeStr=boolean
  PN Sequence Generator : commseqgen2/PN Sequence Generator  poly=scrambler.poly  ini_sta=scrambler.init  outBitMaskSource=Dialog parameter  shift=9  outVarSiz=off  maxOutSizeMode=Dialog parameter  maxOutSize=[10 1]  Ts=scrambler.sdc.pn_samplerate  frameBased=on  sampPerFrame=sdc.Nmb_input_bits  reset=on  bitPackedOutputs=off  outDataType=boolean  numPackedBits=8  bitPackDataSigned=off  bitPackedOutDType=double
  Out1 : Outport
  wires:
  In1/1 -> Data Type Conversion1/1
  Data Type Conversion1/1 -> Logical Operator/2
  Data Type Conversion/1 -> Frame Conversion/1
  Frame Conversion/1 -> Out1/1
  Constant/1 -> PN Sequence Generator/1
  PN Sequence Generator/1 -> Logical Operator/1
  Logical Operator/1 -> Data Type Conversion/1

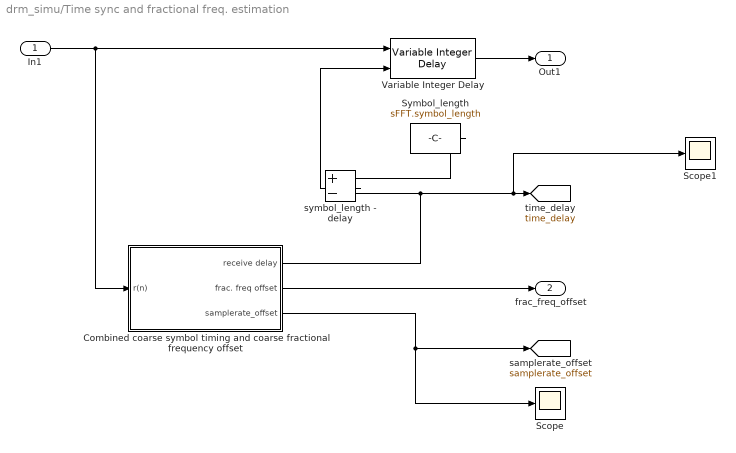
== system drm_simu/Time sync and fractional freq. estimation ==
  In1 : Inport
  Combined coarse symbol timing and coarse fractional frequency offset : Subsystem
  Scope : Scope
  Scope1 : Scope
  Symbol_length : Constant  Value=sFFT.symbol_length
  Variable Integer Delay : dspobslib/Variable Integer Delay  dmax=sFFT.symbol_length  InputProcessing=Inherited (this choice will be removed - see release notes)  ic=0  noDFT=off
  "symbol_length - delay " : Sum  Inputs=+-
  Out1 : Outport
  frac_freq_offset : Outport  Port=2
  tag scope: samplerate_offset=global, time_delay=global
  wires:
  Symbol_length/1 -> "symbol_length - delay "/1
  Combined coarse symbol timing and coarse fractional frequency offset/1(receive delay) -> "symbol_length - delay "/2, Scope1/1, [time_delay]
  In1/1 -> Combined coarse symbol timing and coarse fractional frequency offset/1(r(n)), Variable Integer Delay/1
  "symbol_length - delay "/1 -> Variable Integer Delay/2
  Combined coarse symbol timing and coarse fractional frequency offset/3(samplerate_offset) -> [samplerate_offset], Scope/1
  Combined coarse symbol timing and coarse fractional frequency offset/2(frac. freq offset) -> frac_freq_offset/1
  Variable Integer Delay/1 -> Out1/1

== system drm_simu/demodulator ==
  In1 : Inport
  Downsampling : Subsystem
  IF Demodulator : Subsystem
  Receiver Baseband Spectrum : SpectrumAnalyzer
  Receiver Oversampled Spectrum : SpectrumAnalyzer
  Receiver  IF-Spectrum : SpectrumAnalyzer
  Out1 : Outport
  wires:
  In1/1 -> IF Demodulator/1(s^(t)), Receiver  IF-Spectrum/1
  IF Demodulator/1(g^(t)) -> Downsampling/1(In1), Receiver Oversampled Spectrum/1
  Downsampling/1(Out1) -> Out1/1, Receiver Baseband Spectrum/1

== system drm_simu/modulator ==
  In1 : Inport
  Baseband Spectrum : SpectrumAnalyzer
  IF Spectrum : SpectrumAnalyzer
  IF Modulator : Subsystem
  Oversampled Spectrum : SpectrumAnalyzer
  Upsampling : Subsystem
  Out1 : Outport
  wires:
  Upsampling/1(Out1) -> IF Modulator/1(s_b(t)), Oversampled Spectrum/1
  IF Modulator/1(s(t)) -> Out1/1, IF Spectrum/1
  In1/1 -> Upsampling/1(In1), Baseband Spectrum/1

== system drm_simu/pilot generator ==
  Abs : Abs
  Add all pilots of one frame : Sum  Inputs=+++
  Math Function : Math  Operator=transpose  SaturateOnIntegerOverflow=on
  Pilot positions : dspsnks4/Matrix Viewer  ImageParams=off  CMapStr=jet(256)  AxisColorbar=off  AxisParams=off  AxisOrigin=Upper left corner  XLabel=carrier k  YLabel=symbol s  ZLabel=abs  FigPos=get(0,'defaultfigureposition')  AxisZoom=off
      settings: YMin=0  YMax=2
  "frequency pilots (Frequency reference matrix) " : Constant  Value=ofdm.freq_ref_array  VectorParams1D=off
      settings: SamplingMode=Frame based
  gain pilots (Gain reference matrix) : Constant  Value=ofdm.gain_ref_array  VectorParams1D=off
      settings: SamplingMode=Frame based
  time pilots (Time reference matrix) : Constant  Value=ofdm.time_ref_array  VectorParams1D=off
      settings: SamplingMode=Frame based
  pilot cells : Outport
  wires:
  "frequency pilots (Frequency reference matrix) "/1 -> Add all pilots of one frame/1
  time pilots (Time reference matrix)/1 -> Add all pilots of one frame/2
  gain pilots (Gain reference matrix)/1 -> Add all pilots of one frame/3
  Add all pilots of one frame/1 -> pilot cells/1, Abs/1
  Abs/1 -> Math Function/1
  Math Function/1 -> Pilot positions/1

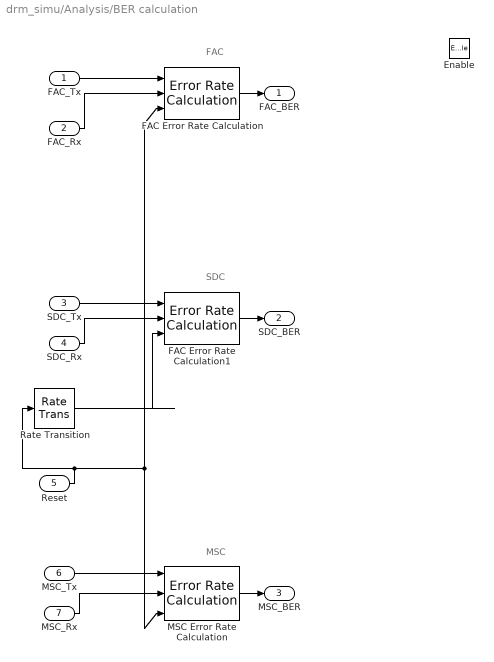
== system drm_simu/Analysis/BER calculation ==
  note: SDC
  note: MSC
  note: FAC
  FAC_Tx : Inport
  FAC_Rx : Inport  Port=2
  SDC_Tx : Inport  Port=3
  SDC_Rx : Inport  Port=4
  Reset : Inport  Port=5
  MSC_Tx : Inport  Port=6
  MSC_Rx : Inport  Port=7
  Enable : EnablePort
  FAC Error Rate Calculation : commsink2/Error Rate Calculation  N=fac.tx_rx_delay  st_delay=0  cp_mode=Entire frame  subframe=[]  PMode=Port  WsName=ErrorVec  RsMode2=on  stop=off  numErr=100  maxBits=1e6
  FAC Error Rate Calculation1 : commsink2/Error Rate Calculation  N=sdc.tx_rx_delay  st_delay=0  cp_mode=Entire frame  subframe=[]  PMode=Port  WsName=ErrorVec  RsMode2=on  stop=off  numErr=100  maxBits=1e6
  MSC Error Rate Calculation : commsink2/Error Rate Calculation  N=msc.tx_rx_delay  st_delay=0  cp_mode=Entire frame  subframe=[]  PMode=Port  WsName=ErrorVec  RsMode2=on  stop=off  numErr=100  maxBits=1e6
  Rate Transition : RateTransition
  FAC_BER : Outport
  SDC_BER : Outport  Port=2
  MSC_BER : Outport  Port=3
  wires:
  Rate Transition/1 -> FAC Error Rate Calculation1/3
  FAC_Tx/1 -> FAC Error Rate Calculation/1
  FAC_Rx/1 -> FAC Error Rate Calculation/2
  FAC Error Rate Calculation/1 -> FAC_BER/1
  SDC_Tx/1 -> FAC Error Rate Calculation1/1
  SDC_Rx/1 -> FAC Error Rate Calculation1/2
  FAC Error Rate Calculation1/1 -> SDC_BER/1
  Reset/1 -> Rate Transition/1, MSC Error Rate Calculation/3, FAC Error Rate Calculation/3
  MSC_Tx/1 -> MSC Error Rate Calculation/1
  MSC_Rx/1 -> MSC Error Rate Calculation/2
  MSC Error Rate Calculation/1 -> MSC_BER/1

== system drm_simu/Analysis/FAC CRC check ==
  Frame Conversion : FrameConversion  InheritSamplingMode=off  OutFrame=Sample-based
  Logical Operator1 : Logic  Operator=NOT  AllPortsSameDT=off  OutDataTypeStr=boolean
  EnBER : Outport
  wires:
  [FAC_checksum] -> Logical Operator1/1
  Frame Conversion/1 -> EnBER/1
  Logical Operator1/1 -> Frame Conversion/1

== system drm_simu/FAC channel coder/Encoder ==
  In1 : Inport
  Convolutional Encoder : commcnvcod2/Convolutional Encoder  trellis=conv_poly  opMode=Terminate trellis by appending bits  DelayedResetAction=off  hasIniStPort=off  hasFinStPort=off  usePuncVector=off  punctureVector=punc_rp35  reset=Unused parameter value
  Puncturing pattern : commsequence2/Puncture  punctureVector=fac.punc_pat0
  Out1 : Outport
  wires:
  Convolutional Encoder/1 -> Puncturing pattern/1
  In1/1 -> Convolutional Encoder/1
  Puncturing pattern/1 -> Out1/1

== system drm_simu/FAC channel decoder/Decoder ==
  In1 : Inport
  Converter for  unquantized decision : commutil2/Unipolar to Bipolar Converter  M=2  polarity=Negative  dataType=Inherit via internal rule
  Depuncture C1 : commsequence2/Insert Zero  insertZeroVector=fac.punc_pat0
  Remove tailbits : dspmtrx3/Submatrix  RowSpan=Range of rows  RowStartMode=First  RowStartIndex=1  RowEndMode=Offset from last  RowEndIndex=6  ColSpan=All columns  ColStartMode=First  ColStartIndex=1  ColEndMode=Last  ColEndIndex=1
  Viterbi Decoder : commcnvcod2/Viterbi Decoder  trellis=conv_poly  isPunctured=off  punctureVector=fac.punc_pat  erasures=off  dectype=Unquantized  runSigValErrCheck=on  nsdecb=3  smWordLength=16  tbdepth=34  opmode=Terminated  reset=off  outDataType=Inherit via internal rule  delayedResetAction=off
  Out1 : Outport
  wires:
  Viterbi Decoder/1 -> Remove tailbits/1
  Depuncture C1/1 -> Viterbi Decoder/1
  Converter for  unquantized decision/1 -> Depuncture C1/1
  In1/1 -> Converter for  unquantized decision/1
  Remove tailbits/1 -> Out1/1

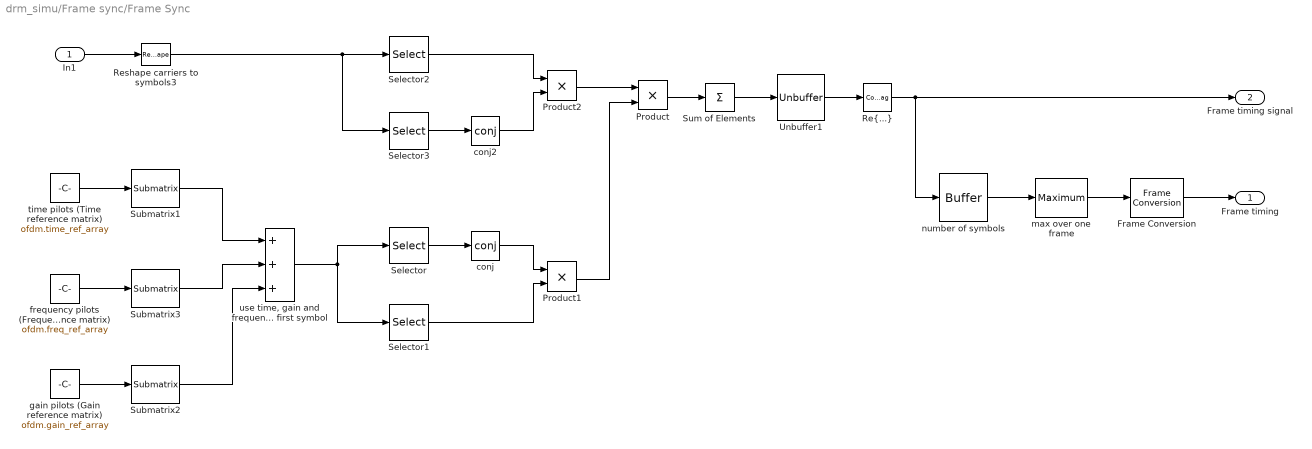
== system drm_simu/Frame sync/Frame Sync ==
  In1 : Inport
  Frame Conversion : FrameConversion  InheritSamplingMode=off  OutFrame=Sample-based
  Product : Product  RndMeth=Zero
  Product1 : Product  RndMeth=Zero
  Product2 : Product  RndMeth=Zero
  Reshape carriers to symbols3 : Reshape  OutputDimensionality=Column vector (2-D)  OutputDimensions=[ofdm.nmb_carriers,ofdm.nmb_symbols]
  "Re{...}" : ComplexToRealImag  Output=Real
  Selector : Selector  InputPortWidth=ofdm.nmb_carriers  IndexOptions=Index vector (dialog)  Indices=sync.pilot_pairs  OutputSizes=1
  Selector1 : Selector  InputPortWidth=ofdm.nmb_carriers  IndexOptions=Index vector (dialog)  Indices=sync.pilot_pairs+1  OutputSizes=1
  Selector2 : Selector  InputPortWidth=ofdm.nmb_carriers  IndexOptions=Index vector (dialog)  Indices=sync.pilot_pairs  OutputSizes=1
  Selector3 : Selector  InputPortWidth=ofdm.nmb_carriers  IndexOptions=Index vector (dialog)  Indices=sync.pilot_pairs+1  OutputSizes=1
  Submatrix1 : dspmtrx3/Submatrix  RowSpan=All rows  RowStartMode=First  RowStartIndex=1  RowEndMode=Index  RowEndIndex=15  ColSpan=Range of columns  ColStartMode=First  ColStartIndex=1  ColEndMode=Index  ColEndIndex=1
  Submatrix2 : dspmtrx3/Submatrix  RowSpan=All rows  RowStartMode=First  RowStartIndex=1  RowEndMode=Index  RowEndIndex=15  ColSpan=Range of columns  ColStartMode=First  ColStartIndex=1  ColEndMode=Index  ColEndIndex=1
  Submatrix3 : dspmtrx3/Submatrix  RowSpan=All rows  RowStartMode=First  RowStartIndex=1  RowEndMode=Index  RowEndIndex=15  ColSpan=Range of columns  ColStartMode=First  ColStartIndex=1  ColEndMode=Index  ColEndIndex=1
  Sum of Elements : Sum  Inputs=+
  Unbuffer1 : Unbuffer
  conj : Math  Operator=conj  SaturateOnIntegerOverflow=on
  conj2 : Math  Operator=conj  SaturateOnIntegerOverflow=on
  "frequency pilots (Frequency reference matrix) " : Constant  Value=ofdm.freq_ref_array  VectorParams1D=off
      settings: SamplingMode=Frame based
  gain pilots (Gain reference matrix) : Constant  Value=ofdm.gain_ref_array  VectorParams1D=off
      settings: SamplingMode=Frame based
  max over one frame : dspstat3/Maximum  fcn=Index  reset=None  InputProcessing=Columns as channels (frame based)  indexBase=Zero  operateOver=Each column  Dimension=1  operation=maximum  roiEnable=off  roiType=Rectangles  roiPortion=Entire ROI  roiOutput=Individual statistics for each ROI  roiFlag=off  accumDataTypeStr=Inherit: Same as product output  accumLastDataTypeStr=Inherit: Same as product output  roundingMode=Floor  overflowMode=off
  number of symbols : Buffer  N=ofdm.nmb_symbols
  time pilots (Time reference matrix) : Constant  Value=ofdm.time_ref_array  VectorParams1D=off
      settings: SamplingMode=Frame based
  "use time, gain and frequency cells of first symbol" : Sum  Inputs=+++
  Frame timing : Outport
  Frame timing signal : Outport  Port=2
  wires:
  time pilots (Time reference matrix)/1 -> Submatrix1/1
  Sum of Elements/1 -> Unbuffer1/1
  In1/1 -> Reshape carriers to symbols3/1
  gain pilots (Gain reference matrix)/1 -> Submatrix2/1
  "use time, gain and frequency cells of first symbol"/1 -> Selector/1, Selector1/1
  Product/1 -> Sum of Elements/1
  "Re{...}"/1 -> number of symbols/1, Frame timing signal/1
  Submatrix1/1 -> "use time, gain and frequency cells of first symbol"/1
  "frequency pilots (Frequency reference matrix) "/1 -> Submatrix3/1
  Submatrix3/1 -> "use time, gain and frequency cells of first symbol"/2
  Selector1/1 -> Product1/2
  Product1/1 -> Product/2
  Selector/1 -> conj/1
  conj/1 -> Product1/1
  Reshape carriers to symbols3/1 -> Selector2/1, Selector3/1
  Selector3/1 -> conj2/1
  Product2/1 -> Product/1
  Selector2/1 -> Product2/1
  conj2/1 -> Product2/2
  Unbuffer1/1 -> "Re{...}"/1
  max over one frame/1 -> Frame Conversion/1
  number of symbols/1 -> max over one frame/1
  Frame Conversion/1 -> Frame timing/1
  Submatrix2/1 -> "use time, gain and frequency cells of first symbol"/3

== system drm_simu/Integer freq. estimation and frequency sync./FFT ==
  In1 : Inport
  FFT : MATLABFcn  MATLABFcn=fft  Output1D=off
  Remove guard interval : dspmtrx3/Submatrix  RowSpan=Range of rows  RowStartMode=Index  RowStartIndex=sFFT.guard_size+1  RowEndMode=Last  RowEndIndex=sFFT.symbol_length  ColSpan=All columns  ColStartMode=First  ColStartIndex=1  ColEndMode=Last  ColEndIndex=1
  Shift back carriers : Selector  NumberOfDimensions=2  InputPortWidth=3  IndexOptions=Index vector (dialog),Select all  Indices=sFFT.backshift_vec,1  OutputSizes=1,1
  Out1 : Outport
  wires:
  In1/1 -> Remove guard interval/1
  Remove guard interval/1 -> FFT/1
  FFT/1 -> Shift back carriers/1
  Shift back carriers/1 -> Out1/1

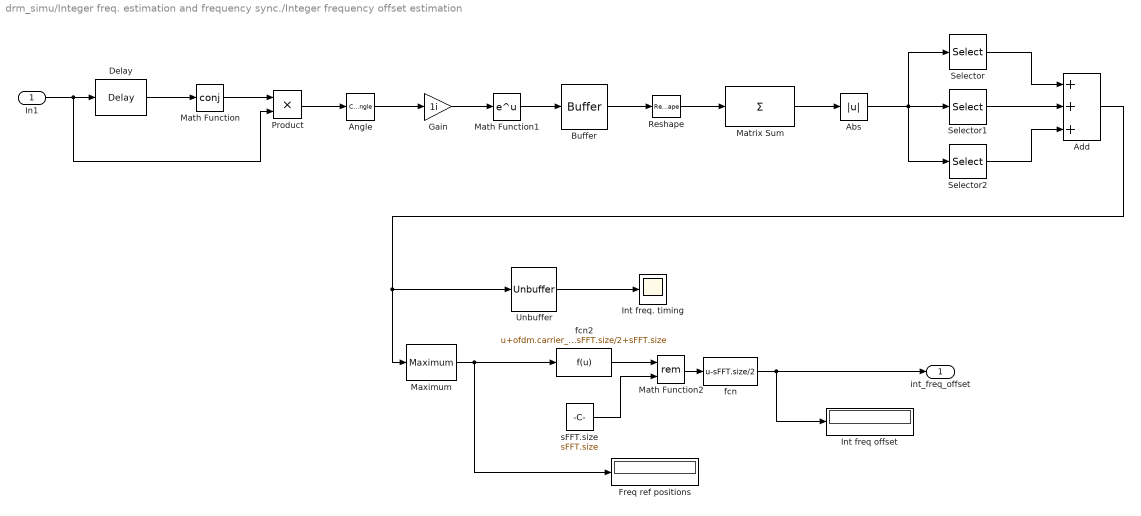
== system drm_simu/Integer freq. estimation and frequency sync./Integer frequency offset estimation ==
  In1 : Inport
  Abs : Abs
  Add : Sum  Inputs=+++
  Angle : ComplexToMagnitudeAngle  Output=Angle
  Buffer : Buffer  N=sFFT.size*ofdm.nmb_symbols
  Delay : dspobslib/Delay  InputProcessing=Inherited (this choice will be removed - see release notes)  dly_unit=Samples  delay=sFFT.size  ic_detail=off  dif_ic_for_ch=off  dif_ic_for_dly=off  ic=0  reset_popup=None
  Freq ref positions : Display
  Gain : Gain  Gain=1i
  Int freq offset : Display
  Int freq. timing : Scope
  Math Function : Math  Operator=conj  SaturateOnIntegerOverflow=on
  Math Function1 : Math  SaturateOnIntegerOverflow=on
  Math Function2 : Math  Operator=rem  SaturateOnIntegerOverflow=on
  Matrix Sum : Sum  Inputs=+  CollapseMode=Specified dimension  CollapseDim=2
  Maximum : dspstat3/Maximum  fcn=Index  reset=None  InputProcessing=Columns as channels (frame based)  indexBase=One  operateOver=Each column  Dimension=1  operation=maximum  roiEnable=off  roiType=Rectangles  roiPortion=Entire ROI  roiOutput=Individual statistics for each ROI  roiFlag=off  accumDataTypeStr=Inherit: Same as product output  accumLastDataTypeStr=Inherit: Same as product output  roundingMode=Floor  overflowMode=off
  Product : Product  RndMeth=Zero
  Reshape : Reshape  OutputDimensionality=Customize  OutputDimensions=[sFFT.size,ofdm.nmb_symbols]
  Selector : Selector  InputPortWidth=sFFT.size  IndexOptions=Select all  Indices=[sync.freq_ref_index(1)+1:sFFT.size 1:sync.freq_ref_index(1)]  OutputSizes=1
  Selector1 : Selector  InputPortWidth=sFFT.size  IndexOptions=Select all  Indices=[sync.freq_ref_index(2)+1:sFFT.size 1:sync.freq_ref_index(2)]  OutputSizes=1
  Selector2 : Selector  InputPortWidth=sFFT.size  IndexOptions=Select all  Indices=[sync.freq_ref_index(3)+1:sFFT.size 1:sync.freq_ref_index(3)]  OutputSizes=1
  Unbuffer : Unbuffer
  fcn : Fcn  Expr=u-sFFT.size/2
  fcn2 : Fcn  Expr=u+ofdm.carrier_min-1+sFFT.size/2+sFFT.size
  sFFT.size : Constant  Value=sFFT.size
  int_freq_offset : Outport
  wires:
  In1/1 -> Delay/1, Product/2
  Delay/1 -> Math Function/1
  Math Function/1 -> Product/1
  Product/1 -> Angle/1
  Angle/1 -> Gain/1
  Gain/1 -> Math Function1/1
  Math Function1/1 -> Buffer/1
  Buffer/1 -> Reshape/1
  Matrix Sum/1 -> Abs/1
  Reshape/1 -> Matrix Sum/1
  Abs/1 -> Selector/1, Selector2/1, Selector1/1
  Selector/1 -> Add/1
  Selector2/1 -> Add/3
  Selector1/1 -> Add/2
  Maximum/1 -> Freq ref positions/1, fcn2/1
  Unbuffer/1 -> Int freq. timing/1
  Add/1 -> Unbuffer/1, Maximum/1
  fcn2/1 -> Math Function2/1
  Math Function2/1 -> fcn/1
  sFFT.size/1 -> Math Function2/2
  fcn/1 -> Int freq offset/1, int_freq_offset/1
